simulink subsystem "ApplicationOpenLoopHighPrio"  (R2024b)
settings: Solver=VariableStepAuto  StartTime=0.0  StopTime=10.0  RelTol=1e-3
libraries: mcbcontrolslib x1, mcbpmsmvflib x1
settings Model: Creator=The MathWorks, Inc.  LastModifiedBy=snarayan
settings RTWCC: GPUComputeCapability=3.5  LargeConstantGeneration=WriteOnlyDNNConstantsToDataFiles

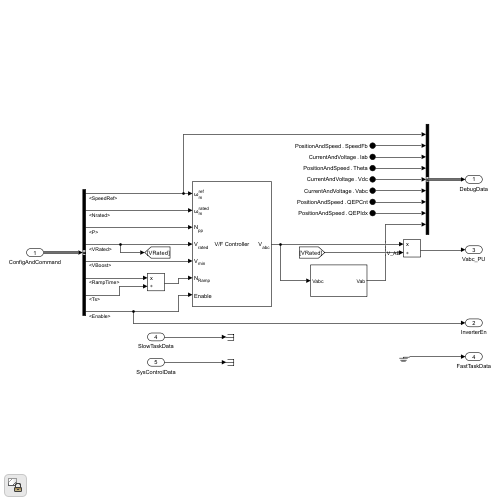
[thumbnail: Simulink's stored preview of the top-level diagram]
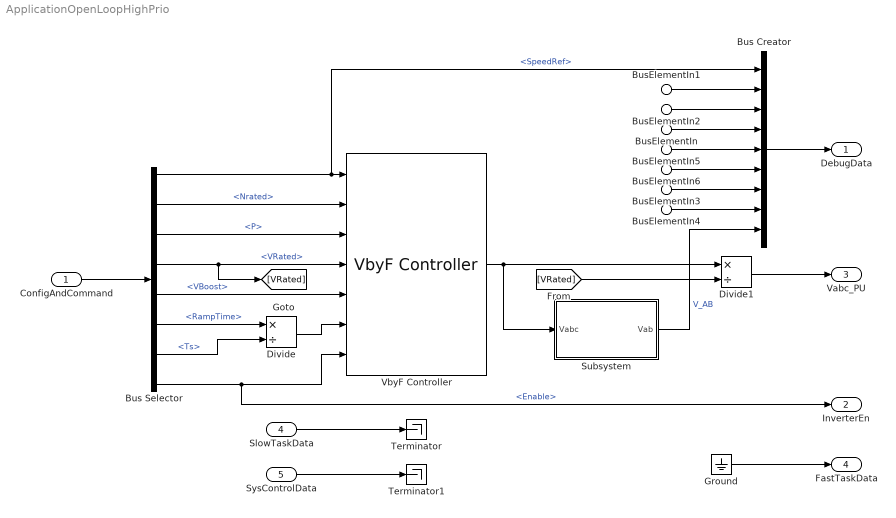
== system ApplicationOpenLoopHighPrio ==
  ConfigAndCommand : Inport
  BusElementIn2 : Inport  Port=2  PortName=CurrentAndVoltage  Element=Iab
  BusElementIn5 : Inport  Port=2  PortName=CurrentAndVoltage  Element=Vdc
  BusElementIn6 : Inport  Port=2  PortName=CurrentAndVoltage  Element=Vabc
  BusElementIn : Inport  Port=3  PortName=PositionAndSpeed  Element=Theta
  BusElementIn1 : Inport  Port=3  PortName=PositionAndSpeed  Element=SpeedFb
  BusElementIn4 : Inport  Port=3  PortName=PositionAndSpeed  Element=QEPIdx
  BusElementIn3 : Inport  Port=3  PortName=PositionAndSpeed  Element=QEPCnt
  SlowTaskData : Inport  Port=4
  SysControlData : Inport  Port=5
  Bus Creator : BusCreator  Inputs=9
  Bus Selector : BusSelector  OutputSignals=SpeedRef,Nrated,P,VRated,VBoost,RampTime,Ts,Enable
  Divide : Product  Inputs=*/  RndMeth=Simplest  OutDataTypeStr=Inherit: Same as first input
  Divide1 : Product  Inputs=*/  RndMeth=Simplest  OutDataTypeStr=Inherit: Same as first input
  Ground : Ground
  Subsystem : Subsystem
  Terminator : Terminator
  Terminator1 : Terminator
  VbyF Controller : mcbpmsmvflib/VbyF Controller  SpeedUnit=RPM  BaseSpeed=1200  Ts=-1
      settings: LibrarySourceBlock=mcblib/Controls/Controllers/VbyF Controller
  DebugData : Outport
  InverterEn : Outport  Port=2
  Vabc_PU : Outport  Port=3
  FastTaskData : Outport  Port=4
  wires:
  SlowTaskData/1 -> Terminator/1
  Divide1/1 -> Vabc_PU/1
  Bus Selector/3 -> VbyF Controller/3  "<P>"
  Bus Selector/6 -> Divide/1  "<RampTime>"
  Bus Selector/7 -> Divide/2  "<Ts>"
  VbyF Controller/1 -> Divide1/1, Subsystem/1(Vabc)
  Bus Creator/1 -> DebugData/1
  ConfigAndCommand/1 -> Bus Selector/1
  Bus Selector/2 -> VbyF Controller/2  "<Nrated>"
  Bus Selector/4 -> VbyF Controller/4, [VRated]  "<VRated>"
  Divide/1 -> VbyF Controller/6
  Bus Selector/5 -> VbyF Controller/5  "<VBoost>"
  SysControlData/1 -> Terminator1/1
  Bus Selector/8 -> VbyF Controller/7, InverterEn/1  "<Enable>"
  Bus Selector/1 -> VbyF Controller/1, Bus Creator/1  "<SpeedRef>"
  [VRated] -> Divide1/2
  Ground/1 -> FastTaskData/1
  BusElementIn1/1 -> Bus Creator/2
  BusElementIn2/1 -> Bus Creator/3
  BusElementIn/1 -> Bus Creator/4
  BusElementIn4/1 -> Bus Creator/8
  BusElementIn3/1 -> Bus Creator/7
  BusElementIn6/1 -> Bus Creator/6
  BusElementIn5/1 -> Bus Creator/5
  Subsystem/1(Vab) -> Bus Creator/9  "V_AB"

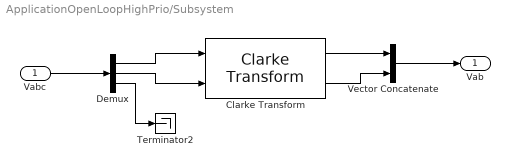
== system ApplicationOpenLoopHighPrio/Subsystem ==
  Vabc : Inport
  Clarke Transform : mcbcontrolslib/Clarke Transform  VariantControl=Variant2  PhaseInput=Two inputs  EnPowerInv=off
      settings: LibrarySourceBlock=mcblib/Controls/Math Transforms/Clarke Transform
  Demux : Demux  Outputs=3
  Terminator2 : Terminator
  Vector Concatenate : Concatenate
  Vab : Outport
  wires:
  Clarke Transform/2 -> Vector Concatenate/2
  Demux/3 -> Terminator2/1
  Demux/2 -> Clarke Transform/2
  Clarke Transform/1 -> Vector Concatenate/1
  Vector Concatenate/1 -> Vab/1
  Demux/1 -> Clarke Transform/1
  Vabc/1 -> Demux/1
